simulink model "sei"  (Simulink 6.2)
settings: Solver=ode45  StartTime=0.0  StopTime=10.0  RelTol=1e-3
libraries: dsparch4 x287, cdsEpicsOut x108, cdsEpicsIn x18, cdsRms x18, Matrix8x x15, cdsSwitch1 x12, cdsProduct x9, Matrix88 x9, cdsSwitch x6, cdsSubtract8 x3, cdsRampSwitch x3, cdsSWD1 x3
(part 4 of 6)

== system sei/HMX_SPARE ==
  In1 : Inport  Port=1  LatchInput=off
  In2 : Inport  Port=2  LatchInput=off
  In3 : Inport  Port=3  LatchInput=off
  In4 : Inport  Port=4  LatchInput=off
  In5 : Inport  Port=5  LatchInput=off
  FP1 : dsparch4/Digital Filter  DialogController=dspDDGCreate  DialogControllerArgs=DataTag157  TypePopup=IIR (poles & zeros)  IIRFiltStruct=Direct form II transposed  AllPoleFiltStruct=Direct form  FIRFiltStruct=Direct form  CoeffSource=Specify via dialog  NumCoeffs=[1 2]  DenCoeffs=[1 0.1]  BiQuadCoeffs=[1 0.3 0.4 1 0.1 0.2]  LatticeCoeffs=[0.2 0.4]  denIgnore=on  FiltPerSampPopup=One filter per frame  IC=0  ICnum=0  ICden=0  roundingMode=Floor  overflowMode=off  ScaleValues=1  scaleValueFracLength=14  stageInFracLength=15  stageOutFracLength=15
  FP2 : dsparch4/Digital Filter  DialogController=dspDDGCreate  DialogControllerArgs=DataTag158  TypePopup=IIR (poles & zeros)  IIRFiltStruct=Direct form II transposed  AllPoleFiltStruct=Direct form  FIRFiltStruct=Direct form  CoeffSource=Specify via dialog  NumCoeffs=[1 2]  DenCoeffs=[1 0.1]  BiQuadCoeffs=[1 0.3 0.4 1 0.1 0.2]  LatticeCoeffs=[0.2 0.4]  denIgnore=on  FiltPerSampPopup=One filter per frame  IC=0  ICnum=0  ICden=0  roundingMode=Floor  overflowMode=off  ScaleValues=1  scaleValueFracLength=14  stageInFracLength=15  stageOutFracLength=15
  RP1 : dsparch4/Digital Filter  DialogController=dspDDGCreate  DialogControllerArgs=DataTag159  TypePopup=IIR (poles & zeros)  IIRFiltStruct=Direct form II transposed  AllPoleFiltStruct=Direct form  FIRFiltStruct=Direct form  CoeffSource=Specify via dialog  NumCoeffs=[1 2]  DenCoeffs=[1 0.1]  BiQuadCoeffs=[1 0.3 0.4 1 0.1 0.2]  LatticeCoeffs=[0.2 0.4]  denIgnore=on  FiltPerSampPopup=One filter per frame  IC=0  ICnum=0  ICden=0  roundingMode=Floor  overflowMode=off  ScaleValues=1  scaleValueFracLength=14  stageInFracLength=15  stageOutFracLength=15
  RP2 : dsparch4/Digital Filter  DialogController=dspDDGCreate  DialogControllerArgs=DataTag160  TypePopup=IIR (poles & zeros)  IIRFiltStruct=Direct form II transposed  AllPoleFiltStruct=Direct form  FIRFiltStruct=Direct form  CoeffSource=Specify via dialog  NumCoeffs=[1 2]  DenCoeffs=[1 0.1]  BiQuadCoeffs=[1 0.3 0.4 1 0.1 0.2]  LatticeCoeffs=[0.2 0.4]  denIgnore=on  FiltPerSampPopup=One filter per frame  IC=0  ICnum=0  ICden=0  roundingMode=Floor  overflowMode=off  ScaleValues=1  scaleValueFracLength=14  stageInFracLength=15  stageOutFracLength=15
  RP3 : dsparch4/Digital Filter  DialogController=dspDDGCreate  DialogControllerArgs=DataTag161  TypePopup=IIR (poles & zeros)  IIRFiltStruct=Direct form II transposed  AllPoleFiltStruct=Direct form  FIRFiltStruct=Direct form  CoeffSource=Specify via dialog  NumCoeffs=[1 2]  DenCoeffs=[1 0.1]  BiQuadCoeffs=[1 0.3 0.4 1 0.1 0.2]  LatticeCoeffs=[0.2 0.4]  denIgnore=on  FiltPerSampPopup=One filter per frame  IC=0  ICnum=0  ICden=0  roundingMode=Floor  overflowMode=off  ScaleValues=1  scaleValueFracLength=14  stageInFracLength=15  stageOutFracLength=15
  Terminator{1..5} (5 alike) : Terminator
  wires:
  RP3/1 -> Terminator5/1
  RP2/1 -> Terminator4/1
  RP1/1 -> Terminator2/1
  FP2/1 -> Terminator1/1
  FP1/1 -> Terminator3/1
  In1/1 -> FP1/1
  In2/1 -> FP2/1
  In3/1 -> RP1/1
  In4/1 -> RP2/1
  In5/1 -> RP3/1

== system sei/HMX_STS ==
  X1 : Inport  Port=1  LatchInput=off
  Y1 : Inport  Port=2  LatchInput=off
  Z1 : Inport  Port=3  LatchInput=off
  X2 : Inport  Port=4  LatchInput=off
  Y2 : Inport  Port=5  LatchInput=off
  Z2 : Inport  Port=6  LatchInput=off
  FIR_X : Inport  Port=7  LatchInput=off
  FIR_Y : Inport  Port=8  LatchInput=off
  IN_MTRX : Matrix88/Subsystem
  MTRX : Matrix88/Subsystem
  RAMP_SW : cdsRampSwitch/Subsystem
  X : dsparch4/Digital Filter  DialogController=dspDDGCreate  DialogControllerArgs=DataTag162  TypePopup=IIR (poles & zeros)  IIRFiltStruct=Direct form II transposed  AllPoleFiltStruct=Direct form  FIRFiltStruct=Direct form  CoeffSource=Specify via dialog  NumCoeffs=[1 2]  DenCoeffs=[1 0.1]  BiQuadCoeffs=[1 0.3 0.4 1 0.1 0.2]  LatticeCoeffs=[0.2 0.4]  denIgnore=on  FiltPerSampPopup=One filter per frame  IC=0  ICnum=0  ICden=0  roundingMode=Floor  overflowMode=off  ScaleValues=1  scaleValueFracLength=14  stageInFracLength=15  stageOutFracLength=15
  X_RY : dsparch4/Digital Filter  DialogController=dspDDGCreate  DialogControllerArgs=DataTag163  TypePopup=IIR (poles & zeros)  IIRFiltStruct=Direct form II transposed  AllPoleFiltStruct=Direct form  FIRFiltStruct=Direct form  CoeffSource=Specify via dialog  NumCoeffs=[1 2]  DenCoeffs=[1 0.1]  BiQuadCoeffs=[1 0.3 0.4 1 0.1 0.2]  LatticeCoeffs=[0.2 0.4]  denIgnore=on  FiltPerSampPopup=One filter per frame  IC=0  ICnum=0  ICden=0  roundingMode=Floor  overflowMode=off  ScaleValues=1  scaleValueFracLength=14  stageInFracLength=15  stageOutFracLength=15
  Y : dsparch4/Digital Filter  DialogController=dspDDGCreate  DialogControllerArgs=DataTag164  TypePopup=IIR (poles & zeros)  IIRFiltStruct=Direct form II transposed  AllPoleFiltStruct=Direct form  FIRFiltStruct=Direct form  CoeffSource=Specify via dialog  NumCoeffs=[1 2]  DenCoeffs=[1 0.1]  BiQuadCoeffs=[1 0.3 0.4 1 0.1 0.2]  LatticeCoeffs=[0.2 0.4]  denIgnore=on  FiltPerSampPopup=One filter per frame  IC=0  ICnum=0  ICden=0  roundingMode=Floor  overflowMode=off  ScaleValues=1  scaleValueFracLength=14  stageInFracLength=15  stageOutFracLength=15
  Y_RX : dsparch4/Digital Filter  DialogController=dspDDGCreate  DialogControllerArgs=DataTag165  TypePopup=IIR (poles & zeros)  IIRFiltStruct=Direct form II transposed  AllPoleFiltStruct=Direct form  FIRFiltStruct=Direct form  CoeffSource=Specify via dialog  NumCoeffs=[1 2]  DenCoeffs=[1 0.1]  BiQuadCoeffs=[1 0.3 0.4 1 0.1 0.2]  LatticeCoeffs=[0.2 0.4]  denIgnore=on  FiltPerSampPopup=One filter per frame  IC=0  ICnum=0  ICden=0  roundingMode=Floor  overflowMode=off  ScaleValues=1  scaleValueFracLength=14  stageInFracLength=15  stageOutFracLength=15
  Z : dsparch4/Digital Filter  DialogController=dspDDGCreate  DialogControllerArgs=DataTag166  TypePopup=IIR (poles & zeros)  IIRFiltStruct=Direct form II transposed  AllPoleFiltStruct=Direct form  FIRFiltStruct=Direct form  CoeffSource=Specify via dialog  NumCoeffs=[1 2]  DenCoeffs=[1 0.1]  BiQuadCoeffs=[1 0.3 0.4 1 0.1 0.2]  LatticeCoeffs=[0.2 0.4]  denIgnore=on  FiltPerSampPopup=One filter per frame  IC=0  ICnum=0  ICden=0  roundingMode=Floor  overflowMode=off  ScaleValues=1  scaleValueFracLength=14  stageInFracLength=15  stageOutFracLength=15
  RX : Outport
  RY : Outport  Port=2
  V1 : Outport  Port=3
  V2 : Outport  Port=4
  V3 : Outport  Port=5
  V4 : Outport  Port=6
  H1 : Outport  Port=7
  H2 : Outport  Port=8
  H3 : Outport  Port=9
  H4 : Outport  Port=10
  WDX : Outport  Port=11
  WDY : Outport  Port=12
  WDZ : Outport  Port=13
  wires:
  IN_MTRX/2 -> Y/1, WDY/1
  IN_MTRX/1 -> X/1, WDX/1
  IN_MTRX/3 -> Z/1, WDZ/1
  Z/1 -> MTRX/3
  X_RY/1 -> RX/1
  Y_RX/1 -> RY/1
  X1/1 -> IN_MTRX/1
  MTRX/1 -> V1/1
  Y1/1 -> IN_MTRX/2
  MTRX/2 -> V2/1
  Z1/1 -> IN_MTRX/3
  MTRX/3 -> V3/1
  X2/1 -> IN_MTRX/4
  MTRX/4 -> V4/1
  Y2/1 -> IN_MTRX/5
  MTRX/5 -> H1/1
  Z2/1 -> IN_MTRX/6
  MTRX/6 -> H2/1
  MTRX/7 -> H3/1
  MTRX/8 -> H4/1
  X/1 -> RAMP_SW/1
  FIR_X/1 -> RAMP_SW/2
  Y/1 -> RAMP_SW/3
  FIR_Y/1 -> RAMP_SW/4
  RAMP_SW/2 -> MTRX/2, Y_RX/1
  RAMP_SW/1 -> MTRX/1, X_RY/1

== system sei/HMX_WD ==
  In1 : Inport  Port=1  LatchInput=off
  In2 : Inport  Port=2  LatchInput=off
  In3 : Inport  Port=3  LatchInput=off
  In4 : Inport  Port=4  LatchInput=off
  In5 : Inport  Port=5  LatchInput=off
  In6 : Inport  Port=6  LatchInput=off
  In7 : Inport  Port=7  LatchInput=off
  In8 : Inport  Port=8  LatchInput=off
  In9 : Inport  Port=9  LatchInput=off
  In10 : Inport  Port=10  LatchInput=off
  In11 : Inport  Port=11  LatchInput=off
  In12 : Inport  Port=12  LatchInput=off
  In13 : Inport  Port=13  LatchInput=off
  In14 : Inport  Port=14  LatchInput=off
  In15 : Inport  Port=15  LatchInput=off
  In16 : Inport  Port=16  LatchInput=off
  In17 : Inport  Port=17  LatchInput=off
  In18 : Inport  Port=18  LatchInput=off
  In19 : Inport  Port=19  LatchInput=off
  GEO_H1 : dsparch4/Digital Filter  DialogController=dspDDGCreate  DialogControllerArgs=DataTag167  TypePopup=IIR (poles & zeros)  IIRFiltStruct=Direct form II transposed  AllPoleFiltStruct=Direct form  FIRFiltStruct=Direct form  CoeffSource=Specify via dialog  NumCoeffs=[1 2]  DenCoeffs=[1 0.1]  BiQuadCoeffs=[1 0.3 0.4 1 0.1 0.2]  LatticeCoeffs=[0.2 0.4]  denIgnore=on  FiltPerSampPopup=One filter per frame  IC=0  ICnum=0  ICden=0  roundingMode=Floor  overflowMode=off  ScaleValues=1  scaleValueFracLength=14  stageInFracLength=15  stageOutFracLength=15
  GEO_H2 : dsparch4/Digital Filter  DialogController=dspDDGCreate  DialogControllerArgs=DataTag168  TypePopup=IIR (poles & zeros)  IIRFiltStruct=Direct form II transposed  AllPoleFiltStruct=Direct form  FIRFiltStruct=Direct form  CoeffSource=Specify via dialog  NumCoeffs=[1 2]  DenCoeffs=[1 0.1]  BiQuadCoeffs=[1 0.3 0.4 1 0.1 0.2]  LatticeCoeffs=[0.2 0.4]  denIgnore=on  FiltPerSampPopup=One filter per frame  IC=0  ICnum=0  ICden=0  roundingMode=Floor  overflowMode=off  ScaleValues=1  scaleValueFracLength=14  stageInFracLength=15  stageOutFracLength=15
  GEO_H3 : dsparch4/Digital Filter  DialogController=dspDDGCreate  DialogControllerArgs=DataTag169  TypePopup=IIR (poles & zeros)  IIRFiltStruct=Direct form II transposed  AllPoleFiltStruct=Direct form  FIRFiltStruct=Direct form  CoeffSource=Specify via dialog  NumCoeffs=[1 2]  DenCoeffs=[1 0.1]  BiQuadCoeffs=[1 0.3 0.4 1 0.1 0.2]  LatticeCoeffs=[0.2 0.4]  denIgnore=on  FiltPerSampPopup=One filter per frame  IC=0  ICnum=0  ICden=0  roundingMode=Floor  overflowMode=off  ScaleValues=1  scaleValueFracLength=14  stageInFracLength=15  stageOutFracLength=15
  GEO_H4 : dsparch4/Digital Filter  DialogController=dspDDGCreate  DialogControllerArgs=DataTag170  TypePopup=IIR (poles & zeros)  IIRFiltStruct=Direct form II transposed  AllPoleFiltStruct=Direct form  FIRFiltStruct=Direct form  CoeffSource=Specify via dialog  NumCoeffs=[1 2]  DenCoeffs=[1 0.1]  BiQuadCoeffs=[1 0.3 0.4 1 0.1 0.2]  LatticeCoeffs=[0.2 0.4]  denIgnore=on  FiltPerSampPopup=One filter per frame  IC=0  ICnum=0  ICden=0  roundingMode=Floor  overflowMode=off  ScaleValues=1  scaleValueFracLength=14  stageInFracLength=15  stageOutFracLength=15
  GEO_V1 : dsparch4/Digital Filter  DialogController=dspDDGCreate  DialogControllerArgs=DataTag171  TypePopup=IIR (poles & zeros)  IIRFiltStruct=Direct form II transposed  AllPoleFiltStruct=Direct form  FIRFiltStruct=Direct form  CoeffSource=Specify via dialog  NumCoeffs=[1 2]  DenCoeffs=[1 0.1]  BiQuadCoeffs=[1 0.3 0.4 1 0.1 0.2]  LatticeCoeffs=[0.2 0.4]  denIgnore=on  FiltPerSampPopup=One filter per frame  IC=0  ICnum=0  ICden=0  roundingMode=Floor  overflowMode=off  ScaleValues=1  scaleValueFracLength=14  stageInFracLength=15  stageOutFracLength=15
  GEO_V2 : dsparch4/Digital Filter  DialogController=dspDDGCreate  DialogControllerArgs=DataTag172  TypePopup=IIR (poles & zeros)  IIRFiltStruct=Direct form II transposed  AllPoleFiltStruct=Direct form  FIRFiltStruct=Direct form  CoeffSource=Specify via dialog  NumCoeffs=[1 2]  DenCoeffs=[1 0.1]  BiQuadCoeffs=[1 0.3 0.4 1 0.1 0.2]  LatticeCoeffs=[0.2 0.4]  denIgnore=on  FiltPerSampPopup=One filter per frame  IC=0  ICnum=0  ICden=0  roundingMode=Floor  overflowMode=off  ScaleValues=1  scaleValueFracLength=14  stageInFracLength=15  stageOutFracLength=15
  GEO_V3 : dsparch4/Digital Filter  DialogController=dspDDGCreate  DialogControllerArgs=DataTag173  TypePopup=IIR (poles & zeros)  IIRFiltStruct=Direct form II transposed  AllPoleFiltStruct=Direct form  FIRFiltStruct=Direct form  CoeffSource=Specify via dialog  NumCoeffs=[1 2]  DenCoeffs=[1 0.1]  BiQuadCoeffs=[1 0.3 0.4 1 0.1 0.2]  LatticeCoeffs=[0.2 0.4]  denIgnore=on  FiltPerSampPopup=One filter per frame  IC=0  ICnum=0  ICden=0  roundingMode=Floor  overflowMode=off  ScaleValues=1  scaleValueFracLength=14  stageInFracLength=15  stageOutFracLength=15
  GEO_V4 : dsparch4/Digital Filter  DialogController=dspDDGCreate  DialogControllerArgs=DataTag174  TypePopup=IIR (poles & zeros)  IIRFiltStruct=Direct form II transposed  AllPoleFiltStruct=Direct form  FIRFiltStruct=Direct form  CoeffSource=Specify via dialog  NumCoeffs=[1 2]  DenCoeffs=[1 0.1]  BiQuadCoeffs=[1 0.3 0.4 1 0.1 0.2]  LatticeCoeffs=[0.2 0.4]  denIgnore=on  FiltPerSampPopup=One filter per frame  IC=0  ICnum=0  ICden=0  roundingMode=Floor  overflowMode=off  ScaleValues=1  scaleValueFracLength=14  stageInFracLength=15  stageOutFracLength=15
  M : cdsSWD1/Subsystem
  POS_H1 : dsparch4/Digital Filter  DialogController=dspDDGCreate  DialogControllerArgs=DataTag175  TypePopup=IIR (poles & zeros)  IIRFiltStruct=Direct form II transposed  AllPoleFiltStruct=Direct form  FIRFiltStruct=Direct form  CoeffSource=Specify via dialog  NumCoeffs=[1 2]  DenCoeffs=[1 0.1]  BiQuadCoeffs=[1 0.3 0.4 1 0.1 0.2]  LatticeCoeffs=[0.2 0.4]  denIgnore=on  FiltPerSampPopup=One filter per frame  IC=0  ICnum=0  ICden=0  roundingMode=Floor  overflowMode=off  ScaleValues=1  scaleValueFracLength=14  stageInFracLength=15  stageOutFracLength=15
  POS_H2 : dsparch4/Digital Filter  DialogController=dspDDGCreate  DialogControllerArgs=DataTag176  TypePopup=IIR (poles & zeros)  IIRFiltStruct=Direct form II transposed  AllPoleFiltStruct=Direct form  FIRFiltStruct=Direct form  CoeffSource=Specify via dialog  NumCoeffs=[1 2]  DenCoeffs=[1 0.1]  BiQuadCoeffs=[1 0.3 0.4 1 0.1 0.2]  LatticeCoeffs=[0.2 0.4]  denIgnore=on  FiltPerSampPopup=One filter per frame  IC=0  ICnum=0  ICden=0  roundingMode=Floor  overflowMode=off  ScaleValues=1  scaleValueFracLength=14  stageInFracLength=15  stageOutFracLength=15
  POS_H3 : dsparch4/Digital Filter  DialogController=dspDDGCreate  DialogControllerArgs=DataTag177  TypePopup=IIR (poles & zeros)  IIRFiltStruct=Direct form II transposed  AllPoleFiltStruct=Direct form  FIRFiltStruct=Direct form  CoeffSource=Specify via dialog  NumCoeffs=[1 2]  DenCoeffs=[1 0.1]  BiQuadCoeffs=[1 0.3 0.4 1 0.1 0.2]  LatticeCoeffs=[0.2 0.4]  denIgnore=on  FiltPerSampPopup=One filter per frame  IC=0  ICnum=0  ICden=0  roundingMode=Floor  overflowMode=off  ScaleValues=1  scaleValueFracLength=14  stageInFracLength=15  stageOutFracLength=15
  POS_H4 : dsparch4/Digital Filter  DialogController=dspDDGCreate  DialogControllerArgs=DataTag178  TypePopup=IIR (poles & zeros)  IIRFiltStruct=Direct form II transposed  AllPoleFiltStruct=Direct form  FIRFiltStruct=Direct form  CoeffSource=Specify via dialog  NumCoeffs=[1 2]  DenCoeffs=[1 0.1]  BiQuadCoeffs=[1 0.3 0.4 1 0.1 0.2]  LatticeCoeffs=[0.2 0.4]  denIgnore=on  FiltPerSampPopup=One filter per frame  IC=0  ICnum=0  ICden=0  roundingMode=Floor  overflowMode=off  ScaleValues=1  scaleValueFracLength=14  stageInFracLength=15  stageOutFracLength=15
  POS_V1 : dsparch4/Digital Filter  DialogController=dspDDGCreate  DialogControllerArgs=DataTag179  TypePopup=IIR (poles & zeros)  IIRFiltStruct=Direct form II transposed  AllPoleFiltStruct=Direct form  FIRFiltStruct=Direct form  CoeffSource=Specify via dialog  NumCoeffs=[1 2]  DenCoeffs=[1 0.1]  BiQuadCoeffs=[1 0.3 0.4 1 0.1 0.2]  LatticeCoeffs=[0.2 0.4]  denIgnore=on  FiltPerSampPopup=One filter per frame  IC=0  ICnum=0  ICden=0  roundingMode=Floor  overflowMode=off  ScaleValues=1  scaleValueFracLength=14  stageInFracLength=15  stageOutFracLength=15
  POS_V2 : dsparch4/Digital Filter  DialogController=dspDDGCreate  DialogControllerArgs=DataTag180  TypePopup=IIR (poles & zeros)  IIRFiltStruct=Direct form II transposed  AllPoleFiltStruct=Direct form  FIRFiltStruct=Direct form  CoeffSource=Specify via dialog  NumCoeffs=[1 2]  DenCoeffs=[1 0.1]  BiQuadCoeffs=[1 0.3 0.4 1 0.1 0.2]  LatticeCoeffs=[0.2 0.4]  denIgnore=on  FiltPerSampPopup=One filter per frame  IC=0  ICnum=0  ICden=0  roundingMode=Floor  overflowMode=off  ScaleValues=1  scaleValueFracLength=14  stageInFracLength=15  stageOutFracLength=15
  POS_V3 : dsparch4/Digital Filter  DialogController=dspDDGCreate  DialogControllerArgs=DataTag181  TypePopup=IIR (poles & zeros)  IIRFiltStruct=Direct form II transposed  AllPoleFiltStruct=Direct form  FIRFiltStruct=Direct form  CoeffSource=Specify via dialog  NumCoeffs=[1 2]  DenCoeffs=[1 0.1]  BiQuadCoeffs=[1 0.3 0.4 1 0.1 0.2]  LatticeCoeffs=[0.2 0.4]  denIgnore=on  FiltPerSampPopup=One filter per frame  IC=0  ICnum=0  ICden=0  roundingMode=Floor  overflowMode=off  ScaleValues=1  scaleValueFracLength=14  stageInFracLength=15  stageOutFracLength=15
  POS_V4 : dsparch4/Digital Filter  DialogController=dspDDGCreate  DialogControllerArgs=DataTag182  TypePopup=IIR (poles & zeros)  IIRFiltStruct=Direct form II transposed  AllPoleFiltStruct=Direct form  FIRFiltStruct=Direct form  CoeffSource=Specify via dialog  NumCoeffs=[1 2]  DenCoeffs=[1 0.1]  BiQuadCoeffs=[1 0.3 0.4 1 0.1 0.2]  LatticeCoeffs=[0.2 0.4]  denIgnore=on  FiltPerSampPopup=One filter per frame  IC=0  ICnum=0  ICden=0  roundingMode=Floor  overflowMode=off  ScaleValues=1  scaleValueFracLength=14  stageInFracLength=15  stageOutFracLength=15
  STSX : dsparch4/Digital Filter  DialogController=dspDDGCreate  DialogControllerArgs=DataTag183  TypePopup=IIR (poles & zeros)  IIRFiltStruct=Direct form II transposed  AllPoleFiltStruct=Direct form  FIRFiltStruct=Direct form  CoeffSource=Specify via dialog  NumCoeffs=[1 2]  DenCoeffs=[1 0.1]  BiQuadCoeffs=[1 0.3 0.4 1 0.1 0.2]  LatticeCoeffs=[0.2 0.4]  denIgnore=on  FiltPerSampPopup=One filter per frame  IC=0  ICnum=0  ICden=0  roundingMode=Floor  overflowMode=off  ScaleValues=1  scaleValueFracLength=14  stageInFracLength=15  stageOutFracLength=15
  STSY : dsparch4/Digital Filter  DialogController=dspDDGCreate  DialogControllerArgs=DataTag184  TypePopup=IIR (poles & zeros)  IIRFiltStruct=Direct form II transposed  AllPoleFiltStruct=Direct form  FIRFiltStruct=Direct form  CoeffSource=Specify via dialog  NumCoeffs=[1 2]  DenCoeffs=[1 0.1]  BiQuadCoeffs=[1 0.3 0.4 1 0.1 0.2]  LatticeCoeffs=[0.2 0.4]  denIgnore=on  FiltPerSampPopup=One filter per frame  IC=0  ICnum=0  ICden=0  roundingMode=Floor  overflowMode=off  ScaleValues=1  scaleValueFracLength=14  stageInFracLength=15  stageOutFracLength=15
  STSZ : dsparch4/Digital Filter  DialogController=dspDDGCreate  DialogControllerArgs=DataTag185  TypePopup=IIR (poles & zeros)  IIRFiltStruct=Direct form II transposed  AllPoleFiltStruct=Direct form  FIRFiltStruct=Direct form  CoeffSource=Specify via dialog  NumCoeffs=[1 2]  DenCoeffs=[1 0.1]  BiQuadCoeffs=[1 0.3 0.4 1 0.1 0.2]  LatticeCoeffs=[0.2 0.4]  denIgnore=on  FiltPerSampPopup=One filter per frame  IC=0  ICnum=0  ICden=0  roundingMode=Floor  overflowMode=off  ScaleValues=1  scaleValueFracLength=14  stageInFracLength=15  stageOutFracLength=15
  wires:
  In1/1 -> STSX/1, M/1
  In2/1 -> STSY/1, M/3
  In3/1 -> STSZ/1, M/5
  In4/1 -> POS_V1/1, M/7
  STSX/1 -> M/2
  STSY/1 -> M/4
  STSZ/1 -> M/6
  POS_V1/1 -> M/8
  In5/1 -> POS_V2/1, M/9
  In6/1 -> POS_V3/1, M/11
  In7/1 -> POS_V4/1, M/13
  In8/1 -> POS_H1/1, M/15
  In9/1 -> POS_H2/1, M/17
  In10/1 -> POS_H3/1, M/19
  In11/1 -> POS_H4/1, M/21
  In12/1 -> GEO_V1/1, M/23
  In13/1 -> GEO_V2/1, M/25
  In14/1 -> GEO_V3/1, M/27
  In15/1 -> GEO_V4/1, M/29
  In16/1 -> GEO_H1/1, M/31
  In17/1 -> GEO_H2/1, M/33
  In18/1 -> GEO_H3/1, M/35
  In19/1 -> GEO_H4/1, M/37
  POS_V2/1 -> M/10
  POS_V3/1 -> M/12
  POS_V4/1 -> M/14
  POS_H1/1 -> M/16
  POS_H2/1 -> M/18
  POS_H3/1 -> M/20
  POS_H4/1 -> M/22
  GEO_V1/1 -> M/24
  GEO_V2/1 -> M/26
  GEO_V3/1 -> M/28
  GEO_V4/1 -> M/30
  GEO_H1/1 -> M/32
  GEO_H2/1 -> M/34
  GEO_H3/1 -> M/36
  GEO_H4/1 -> M/38

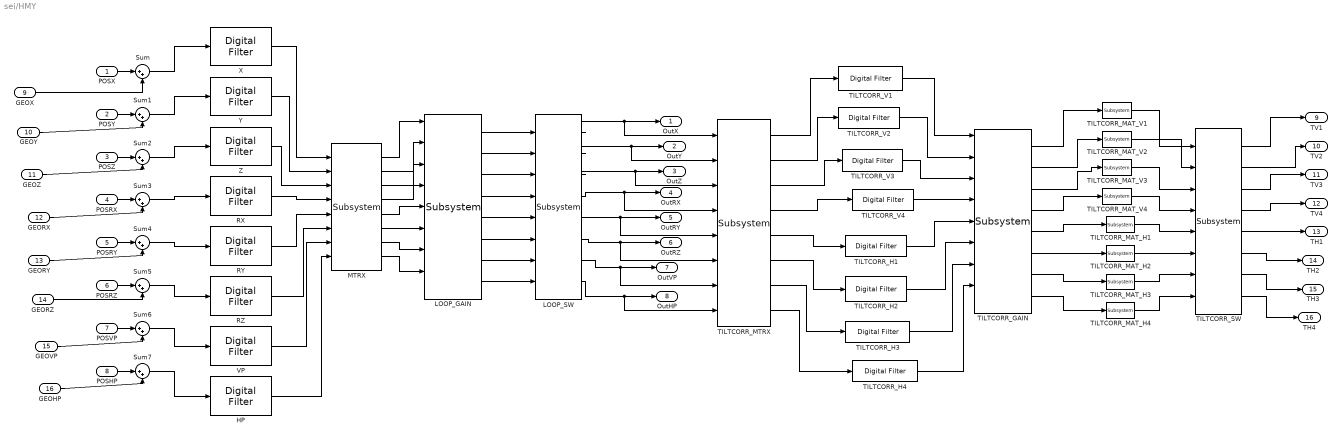
== system sei/HMY ==
  POSX : Inport  Port=1  LatchInput=off
  POSY : Inport  Port=2  LatchInput=off
  POSZ : Inport  Port=3  LatchInput=off
  POSRX : Inport  Port=4  LatchInput=off
  POSRY : Inport  Port=5  LatchInput=off
  POSRZ : Inport  Port=6  LatchInput=off
  POSVP : Inport  Port=7  LatchInput=off
  POSHP : Inport  Port=8  LatchInput=off
  GEOX : Inport  Port=9  LatchInput=off
  GEOY : Inport  Port=10  LatchInput=off
  GEOZ : Inport  Port=11  LatchInput=off
  GEORX : Inport  Port=12  LatchInput=off
  GEORY : Inport  Port=13  LatchInput=off
  GEORZ : Inport  Port=14  LatchInput=off
  GEOVP : Inport  Port=15  LatchInput=off
  GEOHP : Inport  Port=16  LatchInput=off
  HP : dsparch4/Digital Filter  DialogController=dspDDGCreate  DialogControllerArgs=DataTag186  TypePopup=IIR (poles & zeros)  IIRFiltStruct=Direct form II transposed  AllPoleFiltStruct=Direct form  FIRFiltStruct=Direct form  CoeffSource=Specify via dialog  NumCoeffs=[1 2]  DenCoeffs=[1 0.1]  BiQuadCoeffs=[1 0.3 0.4 1 0.1 0.2]  LatticeCoeffs=[0.2 0.4]  denIgnore=on  FiltPerSampPopup=One filter per frame  IC=0  ICnum=0  ICden=0  roundingMode=Floor  overflowMode=off  ScaleValues=1  scaleValueFracLength=14  stageInFracLength=15  stageOutFracLength=15
  LOOP_GAIN : cdsProduct/Subsystem
      settings: AttributesFormatString=%<ReferenceBlock>
  LOOP_SW : cdsSwitch1/Subsystem
      settings: AttributesFormatString=%<ReferenceBlock>
  MTRX : Matrix8x/Subsystem
  RX : dsparch4/Digital Filter  DialogController=dspDDGCreate  DialogControllerArgs=DataTag187  TypePopup=IIR (poles & zeros)  IIRFiltStruct=Direct form II transposed  AllPoleFiltStruct=Direct form  FIRFiltStruct=Direct form  CoeffSource=Specify via dialog  NumCoeffs=[1 2]  DenCoeffs=[1 0.1]  BiQuadCoeffs=[1 0.3 0.4 1 0.1 0.2]  LatticeCoeffs=[0.2 0.4]  denIgnore=on  FiltPerSampPopup=One filter per frame  IC=0  ICnum=0  ICden=0  roundingMode=Floor  overflowMode=off  ScaleValues=1  scaleValueFracLength=14  stageInFracLength=15  stageOutFracLength=15
  RY : dsparch4/Digital Filter  DialogController=dspDDGCreate  DialogControllerArgs=DataTag188  TypePopup=IIR (poles & zeros)  IIRFiltStruct=Direct form II transposed  AllPoleFiltStruct=Direct form  FIRFiltStruct=Direct form  CoeffSource=Specify via dialog  NumCoeffs=[1 2]  DenCoeffs=[1 0.1]  BiQuadCoeffs=[1 0.3 0.4 1 0.1 0.2]  LatticeCoeffs=[0.2 0.4]  denIgnore=on  FiltPerSampPopup=One filter per frame  IC=0  ICnum=0  ICden=0  roundingMode=Floor  overflowMode=off  ScaleValues=1  scaleValueFracLength=14  stageInFracLength=15  stageOutFracLength=15
  RZ : dsparch4/Digital Filter  DialogController=dspDDGCreate  DialogControllerArgs=DataTag189  TypePopup=IIR (poles & zeros)  IIRFiltStruct=Direct form II transposed  AllPoleFiltStruct=Direct form  FIRFiltStruct=Direct form  CoeffSource=Specify via dialog  NumCoeffs=[1 2]  DenCoeffs=[1 0.1]  BiQuadCoeffs=[1 0.3 0.4 1 0.1 0.2]  LatticeCoeffs=[0.2 0.4]  denIgnore=on  FiltPerSampPopup=One filter per frame  IC=0  ICnum=0  ICden=0  roundingMode=Floor  overflowMode=off  ScaleValues=1  scaleValueFracLength=14  stageInFracLength=15  stageOutFracLength=15
  Sum{,1..7} (8 alike) : Sum  Inputs=|++
  TILTCORR_GAIN : cdsProduct/Subsystem
      settings: AttributesFormatString=%<ReferenceBlock>
  TILTCORR_H1 : dsparch4/Digital Filter  DialogController=dspDDGCreate  DialogControllerArgs=DataTag190  TypePopup=IIR (poles & zeros)  IIRFiltStruct=Direct form II transposed  AllPoleFiltStruct=Direct form  FIRFiltStruct=Direct form  CoeffSource=Specify via dialog  NumCoeffs=[1 2]  DenCoeffs=[1 0.1]  BiQuadCoeffs=[1 0.3 0.4 1 0.1 0.2]  LatticeCoeffs=[0.2 0.4]  denIgnore=on  FiltPerSampPopup=One filter per frame  IC=0  ICnum=0  ICden=0  roundingMode=Floor  overflowMode=off  ScaleValues=1  scaleValueFracLength=14  stageInFracLength=15  stageOutFracLength=15
  TILTCORR_H2 : dsparch4/Digital Filter  DialogController=dspDDGCreate  DialogControllerArgs=DataTag191  TypePopup=IIR (poles & zeros)  IIRFiltStruct=Direct form II transposed  AllPoleFiltStruct=Direct form  FIRFiltStruct=Direct form  CoeffSource=Specify via dialog  NumCoeffs=[1 2]  DenCoeffs=[1 0.1]  BiQuadCoeffs=[1 0.3 0.4 1 0.1 0.2]  LatticeCoeffs=[0.2 0.4]  denIgnore=on  FiltPerSampPopup=One filter per frame  IC=0  ICnum=0  ICden=0  roundingMode=Floor  overflowMode=off  ScaleValues=1  scaleValueFracLength=14  stageInFracLength=15  stageOutFracLength=15
  TILTCORR_H3 : dsparch4/Digital Filter  DialogController=dspDDGCreate  DialogControllerArgs=DataTag192  TypePopup=IIR (poles & zeros)  IIRFiltStruct=Direct form II transposed  AllPoleFiltStruct=Direct form  FIRFiltStruct=Direct form  CoeffSource=Specify via dialog  NumCoeffs=[1 2]  DenCoeffs=[1 0.1]  BiQuadCoeffs=[1 0.3 0.4 1 0.1 0.2]  LatticeCoeffs=[0.2 0.4]  denIgnore=on  FiltPerSampPopup=One filter per frame  IC=0  ICnum=0  ICden=0  roundingMode=Floor  overflowMode=off  ScaleValues=1  scaleValueFracLength=14  stageInFracLength=15  stageOutFracLength=15
  TILTCORR_H4 : dsparch4/Digital Filter  DialogController=dspDDGCreate  DialogControllerArgs=DataTag193  TypePopup=IIR (poles & zeros)  IIRFiltStruct=Direct form II transposed  AllPoleFiltStruct=Direct form  FIRFiltStruct=Direct form  CoeffSource=Specify via dialog  NumCoeffs=[1 2]  DenCoeffs=[1 0.1]  BiQuadCoeffs=[1 0.3 0.4 1 0.1 0.2]  LatticeCoeffs=[0.2 0.4]  denIgnore=on  FiltPerSampPopup=One filter per frame  IC=0  ICnum=0  ICden=0  roundingMode=Floor  overflowMode=off  ScaleValues=1  scaleValueFracLength=14  stageInFracLength=15  stageOutFracLength=15
  TILTCORR_MAT_H{1..4} (4 alike) : cdsEpicsOut/Subsystem
  TILTCORR_MAT_V{1..4} (4 alike) : cdsEpicsOut/Subsystem
  TILTCORR_MTRX : Matrix8x/Subsystem
  TILTCORR_SW : cdsSwitch1/Subsystem
      settings: AttributesFormatString=%<ReferenceBlock>
  TILTCORR_V1 : dsparch4/Digital Filter  DialogController=dspDDGCreate  DialogControllerArgs=DataTag194  TypePopup=IIR (poles & zeros)  IIRFiltStruct=Direct form II transposed  AllPoleFiltStruct=Direct form  FIRFiltStruct=Direct form  CoeffSource=Specify via dialog  NumCoeffs=[1 2]  DenCoeffs=[1 0.1]  BiQuadCoeffs=[1 0.3 0.4 1 0.1 0.2]  LatticeCoeffs=[0.2 0.4]  denIgnore=on  FiltPerSampPopup=One filter per frame  IC=0  ICnum=0  ICden=0  roundingMode=Floor  overflowMode=off  ScaleValues=1  scaleValueFracLength=14  stageInFracLength=15  stageOutFracLength=15
  TILTCORR_V2 : dsparch4/Digital Filter  DialogController=dspDDGCreate  DialogControllerArgs=DataTag195  TypePopup=IIR (poles & zeros)  IIRFiltStruct=Direct form II transposed  AllPoleFiltStruct=Direct form  FIRFiltStruct=Direct form  CoeffSource=Specify via dialog  NumCoeffs=[1 2]  DenCoeffs=[1 0.1]  BiQuadCoeffs=[1 0.3 0.4 1 0.1 0.2]  LatticeCoeffs=[0.2 0.4]  denIgnore=on  FiltPerSampPopup=One filter per frame  IC=0  ICnum=0  ICden=0  roundingMode=Floor  overflowMode=off  ScaleValues=1  scaleValueFracLength=14  stageInFracLength=15  stageOutFracLength=15
  TILTCORR_V3 : dsparch4/Digital Filter  DialogController=dspDDGCreate  DialogControllerArgs=DataTag196  TypePopup=IIR (poles & zeros)  IIRFiltStruct=Direct form II transposed  AllPoleFiltStruct=Direct form  FIRFiltStruct=Direct form  CoeffSource=Specify via dialog  NumCoeffs=[1 2]  DenCoeffs=[1 0.1]  BiQuadCoeffs=[1 0.3 0.4 1 0.1 0.2]  LatticeCoeffs=[0.2 0.4]  denIgnore=on  FiltPerSampPopup=One filter per frame  IC=0  ICnum=0  ICden=0  roundingMode=Floor  overflowMode=off  ScaleValues=1  scaleValueFracLength=14  stageInFracLength=15  stageOutFracLength=15
  TILTCORR_V4 : dsparch4/Digital Filter  DialogController=dspDDGCreate  DialogControllerArgs=DataTag197  TypePopup=IIR (poles & zeros)  IIRFiltStruct=Direct form II transposed  AllPoleFiltStruct=Direct form  FIRFiltStruct=Direct form  CoeffSource=Specify via dialog  NumCoeffs=[1 2]  DenCoeffs=[1 0.1]  BiQuadCoeffs=[1 0.3 0.4 1 0.1 0.2]  LatticeCoeffs=[0.2 0.4]  denIgnore=on  FiltPerSampPopup=One filter per frame  IC=0  ICnum=0  ICden=0  roundingMode=Floor  overflowMode=off  ScaleValues=1  scaleValueFracLength=14  stageInFracLength=15  stageOutFracLength=15
  VP : dsparch4/Digital Filter  DialogController=dspDDGCreate  DialogControllerArgs=DataTag198  TypePopup=IIR (poles & zeros)  IIRFiltStruct=Direct form II transposed  AllPoleFiltStruct=Direct form  FIRFiltStruct=Direct form  CoeffSource=Specify via dialog  NumCoeffs=[1 2]  DenCoeffs=[1 0.1]  BiQuadCoeffs=[1 0.3 0.4 1 0.1 0.2]  LatticeCoeffs=[0.2 0.4]  denIgnore=on  FiltPerSampPopup=One filter per frame  IC=0  ICnum=0  ICden=0  roundingMode=Floor  overflowMode=off  ScaleValues=1  scaleValueFracLength=14  stageInFracLength=15  stageOutFracLength=15
  X : dsparch4/Digital Filter  DialogController=dspDDGCreate  DialogControllerArgs=DataTag199  TypePopup=IIR (poles & zeros)  IIRFiltStruct=Direct form II transposed  AllPoleFiltStruct=Direct form  FIRFiltStruct=Direct form  CoeffSource=Specify via dialog  NumCoeffs=[1 2]  DenCoeffs=[1 0.1]  BiQuadCoeffs=[1 0.3 0.4 1 0.1 0.2]  LatticeCoeffs=[0.2 0.4]  denIgnore=on  FiltPerSampPopup=One filter per frame  IC=0  ICnum=0  ICden=0  roundingMode=Floor  overflowMode=off  ScaleValues=1  scaleValueFracLength=14  stageInFracLength=15  stageOutFracLength=15
  Y : dsparch4/Digital Filter  DialogController=dspDDGCreate  DialogControllerArgs=DataTag200  TypePopup=IIR (poles & zeros)  IIRFiltStruct=Direct form II transposed  AllPoleFiltStruct=Direct form  FIRFiltStruct=Direct form  CoeffSource=Specify via dialog  NumCoeffs=[1 2]  DenCoeffs=[1 0.1]  BiQuadCoeffs=[1 0.3 0.4 1 0.1 0.2]  LatticeCoeffs=[0.2 0.4]  denIgnore=on  FiltPerSampPopup=One filter per frame  IC=0  ICnum=0  ICden=0  roundingMode=Floor  overflowMode=off  ScaleValues=1  scaleValueFracLength=14  stageInFracLength=15  stageOutFracLength=15
  Z : dsparch4/Digital Filter  DialogController=dspDDGCreate  DialogControllerArgs=DataTag201  TypePopup=IIR (poles & zeros)  IIRFiltStruct=Direct form II transposed  AllPoleFiltStruct=Direct form  FIRFiltStruct=Direct form  CoeffSource=Specify via dialog  NumCoeffs=[1 2]  DenCoeffs=[1 0.1]  BiQuadCoeffs=[1 0.3 0.4 1 0.1 0.2]  LatticeCoeffs=[0.2 0.4]  denIgnore=on  FiltPerSampPopup=One filter per frame  IC=0  ICnum=0  ICden=0  roundingMode=Floor  overflowMode=off  ScaleValues=1  scaleValueFracLength=14  stageInFracLength=15  stageOutFracLength=15
  OutX : Outport
  OutY : Outport  Port=2
  OutZ : Outport  Port=3
  OutRX : Outport  Port=4
  OutRY : Outport  Port=5
  OutRZ : Outport  Port=6
  OutVP : Outport  Port=7
  OutHP : Outport  Port=8
  TV1 : Outport  Port=9
  TV2 : Outport  Port=10
  TV3 : Outport  Port=11
  TV4 : Outport  Port=12
  TH1 : Outport  Port=13
  TH2 : Outport  Port=14
  TH3 : Outport  Port=15
  TH4 : Outport  Port=16
  wires:
  Sum/1 -> X/1
  Sum1/1 -> Y/1
  Sum2/1 -> Z/1
  Sum3/1 -> RX/1
  Sum4/1 -> RY/1
  Sum5/1 -> RZ/1
  Sum6/1 -> VP/1
  Sum7/1 -> HP/1
  X/1 -> MTRX/1
  Y/1 -> MTRX/2
  Z/1 -> MTRX/3
  RX/1 -> MTRX/4
  RY/1 -> MTRX/5
  RZ/1 -> MTRX/6
  VP/1 -> MTRX/7
  HP/1 -> MTRX/8
  POSX/1 -> Sum/1
  GEOX/1 -> Sum/2
  POSY/1 -> Sum1/1
  GEOY/1 -> Sum1/2
  POSZ/1 -> Sum2/1
  GEOZ/1 -> Sum2/2
  POSRX/1 -> Sum3/1
  GEORX/1 -> Sum3/2
  POSRY/1 -> Sum4/1
  GEORY/1 -> Sum4/2
  POSRZ/1 -> Sum5/1
  GEORZ/1 -> Sum5/2
  POSVP/1 -> Sum6/1
  GEOVP/1 -> Sum6/2
  POSHP/1 -> Sum7/1
  GEOHP/1 -> Sum7/2
  LOOP_GAIN/1 -> LOOP_SW/1
  LOOP_GAIN/2 -> LOOP_SW/2
  LOOP_GAIN/3 -> LOOP_SW/3
  LOOP_GAIN/4 -> LOOP_SW/4
  LOOP_GAIN/5 -> LOOP_SW/5
  LOOP_GAIN/6 -> LOOP_SW/6
  LOOP_GAIN/7 -> LOOP_SW/7
  LOOP_GAIN/8 -> LOOP_SW/8
  LOOP_SW/1 -> OutX/1, TILTCORR_MTRX/1
  LOOP_SW/2 -> OutY/1, TILTCORR_MTRX/2
  LOOP_SW/3 -> OutZ/1, TILTCORR_MTRX/3
  LOOP_SW/4 -> OutRX/1, TILTCORR_MTRX/4
  LOOP_SW/5 -> OutRY/1, TILTCORR_MTRX/5
  LOOP_SW/6 -> OutRZ/1, TILTCORR_MTRX/6
  LOOP_SW/7 -> OutVP/1, TILTCORR_MTRX/7
  LOOP_SW/8 -> OutHP/1, TILTCORR_MTRX/8
  MTRX/1 -> LOOP_GAIN/1
  MTRX/2 -> LOOP_GAIN/2
  MTRX/3 -> LOOP_GAIN/3
  MTRX/4 -> LOOP_GAIN/4
  MTRX/5 -> LOOP_GAIN/5
  MTRX/6 -> LOOP_GAIN/6
  MTRX/7 -> LOOP_GAIN/7
  MTRX/8 -> LOOP_GAIN/8
  TILTCORR_MTRX/1 -> TILTCORR_V1/1
  TILTCORR_MTRX/2 -> TILTCORR_V2/1
  TILTCORR_MTRX/3 -> TILTCORR_V3/1
  TILTCORR_MTRX/4 -> TILTCORR_V4/1
  TILTCORR_MTRX/5 -> TILTCORR_H1/1
  TILTCORR_MTRX/6 -> TILTCORR_H2/1
  TILTCORR_MTRX/7 -> TILTCORR_H3/1
  TILTCORR_MTRX/8 -> TILTCORR_H4/1
  TILTCORR_V1/1 -> TILTCORR_GAIN/1
  TILTCORR_V2/1 -> TILTCORR_GAIN/2
  TILTCORR_V3/1 -> TILTCORR_GAIN/3
  TILTCORR_V4/1 -> TILTCORR_GAIN/4
  TILTCORR_H1/1 -> TILTCORR_GAIN/5
  TILTCORR_H2/1 -> TILTCORR_GAIN/6
  TILTCORR_H3/1 -> TILTCORR_GAIN/7
  TILTCORR_H4/1 -> TILTCORR_GAIN/8
  TILTCORR_GAIN/1 -> TILTCORR_MAT_V1/1
  TILTCORR_GAIN/2 -> TILTCORR_MAT_V2/1
  TILTCORR_GAIN/3 -> TILTCORR_MAT_V3/1
  TILTCORR_GAIN/4 -> TILTCORR_MAT_V4/1
  TILTCORR_GAIN/5 -> TILTCORR_MAT_H1/1
  TILTCORR_GAIN/6 -> TILTCORR_MAT_H2/1
  TILTCORR_GAIN/7 -> TILTCORR_MAT_H3/1
  TILTCORR_GAIN/8 -> TILTCORR_MAT_H4/1
  TILTCORR_MAT_V1/1 -> TILTCORR_SW/1
  TILTCORR_MAT_V2/1 -> TILTCORR_SW/2
  TILTCORR_MAT_V3/1 -> TILTCORR_SW/3
  TILTCORR_MAT_V4/1 -> TILTCORR_SW/4
  TILTCORR_MAT_H1/1 -> TILTCORR_SW/5
  TILTCORR_MAT_H2/1 -> TILTCORR_SW/6
  TILTCORR_MAT_H3/1 -> TILTCORR_SW/7
  TILTCORR_MAT_H4/1 -> TILTCORR_SW/8
  TILTCORR_SW/1 -> TV1/1
  TILTCORR_SW/2 -> TV2/1
  TILTCORR_SW/3 -> TV3/1
  TILTCORR_SW/4 -> TV4/1
  TILTCORR_SW/5 -> TH1/1
  TILTCORR_SW/6 -> TH2/1
  TILTCORR_SW/7 -> TH3/1
  TILTCORR_SW/8 -> TH4/1

== system sei/HMY_ACT ==
  V1In : Inport  Port=1  LatchInput=off
  V2In : Inport  Port=2  LatchInput=off
  V3In : Inport  Port=3  LatchInput=off
  V4In : Inport  Port=4  LatchInput=off
  H1In : Inport  Port=5  LatchInput=off
  H2In : Inport  Port=6  LatchInput=off
  H3In : Inport  Port=7  LatchInput=off
  H4In : Inport  Port=8  LatchInput=off
  V1DC : Inport  Port=9  LatchInput=off
  V2DC : Inport  Port=10  LatchInput=off
  V3DC : Inport  Port=11  LatchInput=off
  V4DC : Inport  Port=12  LatchInput=off
  H1DC : Inport  Port=13  LatchInput=off
  H2DC : Inport  Port=14  LatchInput=off
  H3DC : Inport  Port=15  LatchInput=off
  H4DC : Inport  Port=16  LatchInput=off
  GAIN : cdsProduct/Subsystem
  H1 : dsparch4/Digital Filter  DialogController=dspDDGCreate  DialogControllerArgs=DataTag202  TypePopup=IIR (poles & zeros)  IIRFiltStruct=Direct form II transposed  AllPoleFiltStruct=Direct form  FIRFiltStruct=Direct form  CoeffSource=Specify via dialog  NumCoeffs=[1 2]  DenCoeffs=[1 0.1]  BiQuadCoeffs=[1 0.3 0.4 1 0.1 0.2]  LatticeCoeffs=[0.2 0.4]  denIgnore=on  FiltPerSampPopup=One filter per frame  IC=0  ICnum=0  ICden=0  roundingMode=Floor  overflowMode=off  ScaleValues=1  scaleValueFracLength=14  stageInFracLength=15  stageOutFracLength=15
  H2 : dsparch4/Digital Filter  DialogController=dspDDGCreate  DialogControllerArgs=DataTag203  TypePopup=IIR (poles & zeros)  IIRFiltStruct=Direct form II transposed  AllPoleFiltStruct=Direct form  FIRFiltStruct=Direct form  CoeffSource=Specify via dialog  NumCoeffs=[1 2]  DenCoeffs=[1 0.1]  BiQuadCoeffs=[1 0.3 0.4 1 0.1 0.2]  LatticeCoeffs=[0.2 0.4]  denIgnore=on  FiltPerSampPopup=One filter per frame  IC=0  ICnum=0  ICden=0  roundingMode=Floor  overflowMode=off  ScaleValues=1  scaleValueFracLength=14  stageInFracLength=15  stageOutFracLength=15
  H3 : dsparch4/Digital Filter  DialogController=dspDDGCreate  DialogControllerArgs=DataTag204  TypePopup=IIR (poles & zeros)  IIRFiltStruct=Direct form II transposed  AllPoleFiltStruct=Direct form  FIRFiltStruct=Direct form  CoeffSource=Specify via dialog  NumCoeffs=[1 2]  DenCoeffs=[1 0.1]  BiQuadCoeffs=[1 0.3 0.4 1 0.1 0.2]  LatticeCoeffs=[0.2 0.4]  denIgnore=on  FiltPerSampPopup=One filter per frame  IC=0  ICnum=0  ICden=0  roundingMode=Floor  overflowMode=off  ScaleValues=1  scaleValueFracLength=14  stageInFracLength=15  stageOutFracLength=15
  H4 : dsparch4/Digital Filter  DialogController=dspDDGCreate  DialogControllerArgs=DataTag205  TypePopup=IIR (poles & zeros)  IIRFiltStruct=Direct form II transposed  AllPoleFiltStruct=Direct form  FIRFiltStruct=Direct form  CoeffSource=Specify via dialog  NumCoeffs=[1 2]  DenCoeffs=[1 0.1]  BiQuadCoeffs=[1 0.3 0.4 1 0.1 0.2]  LatticeCoeffs=[0.2 0.4]  denIgnore=on  FiltPerSampPopup=One filter per frame  IC=0  ICnum=0  ICden=0  roundingMode=Floor  overflowMode=off  ScaleValues=1  scaleValueFracLength=14  stageInFracLength=15  stageOutFracLength=15
  SW : cdsSwitch1/Subsystem
  Sum{,1..7} (8 alike) : Sum  Inputs=|++
  V1 : dsparch4/Digital Filter  DialogController=dspDDGCreate  DialogControllerArgs=DataTag206  TypePopup=IIR (poles & zeros)  IIRFiltStruct=Direct form II transposed  AllPoleFiltStruct=Direct form  FIRFiltStruct=Direct form  CoeffSource=Specify via dialog  NumCoeffs=[1 2]  DenCoeffs=[1 0.1]  BiQuadCoeffs=[1 0.3 0.4 1 0.1 0.2]  LatticeCoeffs=[0.2 0.4]  denIgnore=on  FiltPerSampPopup=One filter per frame  IC=0  ICnum=0  ICden=0  roundingMode=Floor  overflowMode=off  ScaleValues=1  scaleValueFracLength=14  stageInFracLength=15  stageOutFracLength=15
  V2 : dsparch4/Digital Filter  DialogController=dspDDGCreate  DialogControllerArgs=DataTag207  TypePopup=IIR (poles & zeros)  IIRFiltStruct=Direct form II transposed  AllPoleFiltStruct=Direct form  FIRFiltStruct=Direct form  CoeffSource=Specify via dialog  NumCoeffs=[1 2]  DenCoeffs=[1 0.1]  BiQuadCoeffs=[1 0.3 0.4 1 0.1 0.2]  LatticeCoeffs=[0.2 0.4]  denIgnore=on  FiltPerSampPopup=One filter per frame  IC=0  ICnum=0  ICden=0  roundingMode=Floor  overflowMode=off  ScaleValues=1  scaleValueFracLength=14  stageInFracLength=15  stageOutFracLength=15
  V3 : dsparch4/Digital Filter  DialogController=dspDDGCreate  DialogControllerArgs=DataTag208  TypePopup=IIR (poles & zeros)  IIRFiltStruct=Direct form II transposed  AllPoleFiltStruct=Direct form  FIRFiltStruct=Direct form  CoeffSource=Specify via dialog  NumCoeffs=[1 2]  DenCoeffs=[1 0.1]  BiQuadCoeffs=[1 0.3 0.4 1 0.1 0.2]  LatticeCoeffs=[0.2 0.4]  denIgnore=on  FiltPerSampPopup=One filter per frame  IC=0  ICnum=0  ICden=0  roundingMode=Floor  overflowMode=off  ScaleValues=1  scaleValueFracLength=14  stageInFracLength=15  stageOutFracLength=15
  V4 : dsparch4/Digital Filter  DialogController=dspDDGCreate  DialogControllerArgs=DataTag209  TypePopup=IIR (poles & zeros)  IIRFiltStruct=Direct form II transposed  AllPoleFiltStruct=Direct form  FIRFiltStruct=Direct form  CoeffSource=Specify via dialog  NumCoeffs=[1 2]  DenCoeffs=[1 0.1]  BiQuadCoeffs=[1 0.3 0.4 1 0.1 0.2]  LatticeCoeffs=[0.2 0.4]  denIgnore=on  FiltPerSampPopup=One filter per frame  IC=0  ICnum=0  ICden=0  roundingMode=Floor  overflowMode=off  ScaleValues=1  scaleValueFracLength=14  stageInFracLength=15  stageOutFracLength=15
  OutV1 : Outport
  OutV2 : Outport  Port=2
  OutV3 : Outport  Port=3
  OutV4 : Outport  Port=4
  OutH1 : Outport  Port=5
  OutH2 : Outport  Port=6
  OutH3 : Outport  Port=7
  OutH4 : Outport  Port=8
  wires:
  GAIN/1 -> SW/1
  GAIN/2 -> SW/2
  GAIN/3 -> SW/3
  GAIN/4 -> SW/4
  GAIN/5 -> SW/5
  GAIN/6 -> SW/6
  GAIN/7 -> SW/7
  GAIN/8 -> SW/8
  V1DC/1 -> Sum/2
  V2DC/1 -> Sum1/2
  V3DC/1 -> Sum2/2
  V4DC/1 -> Sum3/2
  H1DC/1 -> Sum4/2
  H2DC/1 -> Sum5/2
  H3DC/1 -> Sum6/2
  H4DC/1 -> Sum7/2
  Sum4/1 -> H1/1
  Sum5/1 -> H2/1
  Sum6/1 -> H3/1
  Sum7/1 -> H4/1
  Sum3/1 -> V4/1
  Sum2/1 -> V3/1
  Sum1/1 -> V2/1
  Sum/1 -> V1/1
  V1In/1 -> Sum/1
  V2In/1 -> Sum1/1
  V3In/1 -> Sum2/1
  V4In/1 -> Sum3/1
  H1In/1 -> Sum4/1
  H2In/1 -> Sum5/1
  H3In/1 -> Sum6/1
  H4In/1 -> Sum7/1
  V1/1 -> GAIN/1
  V2/1 -> GAIN/2
  V3/1 -> GAIN/3
  V4/1 -> GAIN/4
  H1/1 -> GAIN/5
  H2/1 -> GAIN/6
  H3/1 -> GAIN/7
  H4/1 -> GAIN/8
  SW/1 -> OutV1/1
  SW/2 -> OutV2/1
  SW/3 -> OutV3/1
  SW/4 -> OutV4/1
  SW/5 -> OutH1/1
  SW/6 -> OutH2/1
  SW/7 -> OutH3/1
  SW/8 -> OutH4/1

== system sei/HMY_DC_BIAS ==
  {1..6} (6 alike) : cdsEpicsIn/Subsystem
  MTRX : Matrix8x/Subsystem
  SW : cdsSwitch1/Subsystem
  V1 : Outport
  V2 : Outport  Port=2
  V3 : Outport  Port=3
  V4 : Outport  Port=4
  H1 : Outport  Port=5
  H2 : Outport  Port=6
  H3 : Outport  Port=7
  H4 : Outport  Port=8
  wires:
  1/1 -> MTRX/1
  2/1 -> MTRX/2
  3/1 -> MTRX/3
  4/1 -> MTRX/4
  5/1 -> MTRX/5
  6/1 -> MTRX/6
  MTRX/1 -> SW/1
  MTRX/2 -> SW/2
  MTRX/3 -> SW/3
  MTRX/4 -> SW/4
  MTRX/5 -> SW/5
  MTRX/6 -> SW/6
  MTRX/7 -> SW/7
  MTRX/8 -> SW/8
  SW/1 -> V1/1
  SW/2 -> V2/1
  SW/3 -> V3/1
  SW/4 -> V4/1
  SW/5 -> H1/1
  SW/6 -> H2/1
  SW/7 -> H3/1
  SW/8 -> H4/1

== system sei/HMY_FIR ==
  X1 : Inport  Port=1  LatchInput=off
  Y1 : Inport  Port=2  LatchInput=off
  X2 : Inport  Port=3  LatchInput=off
  Y2 : Inport  Port=4  LatchInput=off
  MTRX : Matrix88/Subsystem
  X_OUT : dsparch4/Digital Filter  DialogController=dspDDGCreate  DialogControllerArgs=DataTag210  TypePopup=IIR (poles & zeros)  IIRFiltStruct=Direct form II transposed  AllPoleFiltStruct=Direct form  FIRFiltStruct=Direct form  CoeffSource=Specify via dialog  NumCoeffs=[1 2]  DenCoeffs=[1 0.1]  BiQuadCoeffs=[1 0.3 0.4 1 0.1 0.2]  LatticeCoeffs=[0.2 0.4]  denIgnore=on  FiltPerSampPopup=One filter per frame  IC=0  ICnum=0  ICden=0  roundingMode=Floor  overflowMode=off  ScaleValues=1  scaleValueFracLength=14  stageInFracLength=15  stageOutFracLength=15
  Y_OUT : dsparch4/Digital Filter  DialogController=dspDDGCreate  DialogControllerArgs=DataTag211  TypePopup=IIR (poles & zeros)  IIRFiltStruct=Direct form II transposed  AllPoleFiltStruct=Direct form  FIRFiltStruct=Direct form  CoeffSource=Specify via dialog  NumCoeffs=[1 2]  DenCoeffs=[1 0.1]  BiQuadCoeffs=[1 0.3 0.4 1 0.1 0.2]  LatticeCoeffs=[0.2 0.4]  denIgnore=on  FiltPerSampPopup=One filter per frame  IC=0  ICnum=0  ICden=0  roundingMode=Floor  overflowMode=off  ScaleValues=1  scaleValueFracLength=14  stageInFracLength=15  stageOutFracLength=15
  X : Outport
  Y : Outport  Port=2
  wires:
  MTRX/1 -> X_OUT/1
  MTRX/2 -> Y_OUT/1
  X1/1 -> MTRX/1
  X_OUT/1 -> X/1
  Y1/1 -> MTRX/2
  X2/1 -> MTRX/3
  Y2/1 -> MTRX/4
  Y_OUT/1 -> Y/1
